simulink library "phaseddetectlib"  (R2015a)
settings: Solver=ode45  StartTime=0.0  StopTime=10.0  RelTol=1e-3
values from neighbouring files (symbols this model uses):
  D = Nsig    [espritdoa.m]    (also in radarvcd.m = sqrt((1 + (2 * zeta ./ sqrt(zeta.^2 + 3)))/3); rootmusicdoa.m = D + conv(noise_eigenvects(:,i),conj(flipud(noise_eigenvects()
undefined symbols (not defined in the file or in its folder): magnitude, physconst
libraries: dspmtrx3 x1, dspsigattribs x1
settings Model: CovSFcnEnable=off  Creator=The MathWorks Inc.  LastModifiedBy=The MathWorks Inc.
settings DebuggingCC: UnderspecifiedInitializationDetection=Classic  MergeDetectMultiDrivingBlocksExec=none  SolverPrmCheckMsg=warning

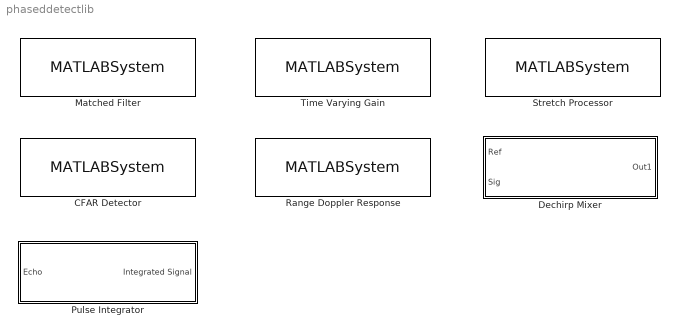
== system phaseddetectlib ==
  CFAR Detector : MATLABSystem  System=phased.CFARDetector  Method=CA  Rank=1  NumGuardCells=2  NumTrainingCells=2  ThresholdFactor=Auto  ProbabilityFalseAlarm=0.1  CustomThresholdFactor=1  ThresholdOutputPort=off  SimulateUsing=Interpreted execution
      mask Type: phased.CFARDetector
      mask Display:
      | disp('CA CFAR');
      | port_label('input',1,'X');
      | port_label('input',2,'Idx');
      | port_label('output',1,'Y');
  Dechirp Mixer : Subsystem  mask(Dechirp){}
      mask help: Mix the input signal with the reference signal. The input signal can be a matrix where each column is a independent channel. The reference signal is a vector. The reference signal is conjugated and then multiplied with each column to compute the output.
      mask Display:
      | port_label('input',1,'RefX');
      | port_label('input',2,'X');
      | port_label('output',1,' ');
      | fprintf('Dechirp')
  Matched Filter : MATLABSystem  System=phased.MatchedFilter  CoefficientsSource=Property  Coefficients=[ 1; 1 ]  SpectrumWindow=None  CustomSpectrumWindow=@hamming  SpectrumRange=[ 0, 1e5 ]  SidelobeAttenuation=30  Beta=0.5  Nbar=4  GainOutputPort=off  SimulateUsing=Interpreted execution
      mask Type: phased.MatchedFilter
      mask Display:
      | disp(['Matched' char(10) 'Filter']);
      | port_label('input',1,'X');
      | port_label('output',1,'Y');
  Pulse Integrator : Subsystem  TreatAsAtomicUnit=on  mask(Pulse Integrator){CoherentFlag=Coherent, N=10, V=0}
      mask prompts: CoherentFlag "Integration method:"; N "Number of pulses to integrate:"; V "Integration overlap (in pulses):"
      mask help: Coherently or noncoherently integrate successive pulses. The input is a column vector representing a pulse. The buffer size, N, specifies how many pulses are integrated. The integration overlap, V, specifies the number of overlapped pulses in successive integrations. V must be less than N.
      mask init:
      | cstr = get_param(gcb,'CoherentFlag');
      | set_param([gcb, '/Integrator'],'OverrideUsingVariant',cstr);
      | validateattributes(N,{'numeric'},{'positive','integer'},'','N');
      | validateattributes(V,{'numeric'},{'integer','>=',0,'<',N},'','K');
      | if strcmp(cstr,'Coherent')
      |     outstr = '\Sigma x';
      | else
      |     outstr = '(\Sigma{|x|^2})^{1/2}';
      | end
      mask TypeOptions CoherentFlag: Coherent | Noncoherent
      mask Display:
      | fprintf('%s\n%d-Pulse\nIntegrator',cstr,N)
      | port_label('input',1,'x');
      | port_label('output',1,outstr,'texmode','on');
  Range Doppler Response : MATLABSystem  System=phased.RangeDopplerResponse  RangeMethod=Matched filter  PropagationSpeed=physconst( 'lightspeed' )  SweepSlope=1e9  DechirpInput=off  RangeFFTLengthSource=Auto  RangeFFTLength=1024  RangeWindow=None  RangeSidelobeAttenuation=30  CustomRangeWindow=@hamming  DopplerFFTLengthSource=Auto  DopplerFFTLength=1024  DopplerWindow=None  DopplerSidelobeAttenuation=30  CustomDopplerWindow=@hamming  DopplerOutput=Frequency  OperatingFrequency=3e8  SimulateUsing=Interpreted execution
      mask Type: phased.RangeDopplerResponse
      mask Display:
      | disp(['Range-Doppler' char(10) 'Response']);
      | port_label('input',1,'X');
      | port_label('input',2,'Coeff');
      | port_label('output',1,'Resp');
      | port_label('output',2,'Range');
      | port_label('output',3,'Dop');
  Stretch Processor : MATLABSystem  System=phased.StretchProcessor  PulseWidth=50e-6  PRF=1e4  SweepSlope=2e9  SweepInterval=Positive  PropagationSpeed=physconst( 'LightSpeed' )  ReferenceRange=5000  RangeSpan=500  SimulateUsing=Interpreted execution
      mask Type: phased.StretchProcessor
      mask Display: disp(['Stretch' char(10) 'Processor']);
  Time Varying Gain : MATLABSystem  System=phased.TimeVaryingGain  RangeLoss=0  ReferenceLoss=0  SimulateUsing=Interpreted execution
      mask Type: phased.TimeVaryingGain
      mask Display: disp('TVG');

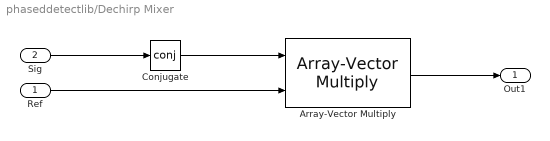
== system phaseddetectlib/Dechirp Mixer ==
  Ref : Inport
  Sig : Inport  Port=2
  Array-Vector Multiply : dspmtrx3/Array-Vector Multiply  mode=Mute  saveAsFlag=0  Dimension=1  V_Source=Input port  V_VectFromMask=[0.5 0.25]  firstCoeffSignedness=Auto  firstCoeffDataTypeStr=Inherit: Same word length as input  firstCoeffLastDataTypeStr=Inherit: Same word length as input  firstCoeffMin=[]  firstCoeffMax=[]  outputSignedness=Auto  outputDataTypeStr=Inherit: Same as product output  outputLastDataTypeStr=Inherit: Same as product output  outputMin=[]  outputMax=[]  accumSignedness=Auto  prodOutputSignedness=Auto  roundingMode=Floor  overflowMode=off
  Conjugate : Math  Operator=conj  SaturateOnIntegerOverflow=on
  Out1 : Outport
  wires:
  Array-Vector Multiply/1 -> Out1/1
  Conjugate/1 -> Array-Vector Multiply/1
  Sig/1 -> Conjugate/1
  Ref/1 -> Array-Vector Multiply/2

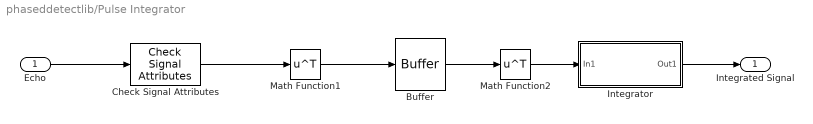
== system phaseddetectlib/Pulse Integrator ==
  Echo : Inport
  Buffer : Buffer  N=N  V=V  TreatMby1Signals=One channel
  Check Signal Attributes : dspsigattribs/Check Signal Attributes  SigAttribCheckMethod=Does not match attributes exactly  Complexity=Ignore  Frame=Ignore  DimsCheckMethod=Is...  Dimensions=Column vector (2-D) or scalar  DatatypeCheckMethod=Ignore  DatatypeGeneral=Boolean  DtypeFloatSpecific=Any floating-point  DtypeFixedSpecific=Any fixed-point  DtypeIntSpecific=Any integer  SampleMode=Ignore
  Integrator : Subsystem  Variant=on  OverrideUsingVariant=Coherent
  Math Function1 : Math  Operator=transpose  OutputSignalType=complex  SaturateOnIntegerOverflow=on
  Math Function2 : Math  Operator=transpose  OutputSignalType=complex  SaturateOnIntegerOverflow=on
  Integrated Signal : Outport
  wires:
  Buffer/1 -> Math Function2/1
  Echo/1 -> Check Signal Attributes/1
  Math Function1/1 -> Buffer/1
  Math Function2/1 -> Integrator/1(In1)
  Integrator/1(Out1) -> Integrated Signal/1
  Check Signal Attributes/1 -> Math Function1/1

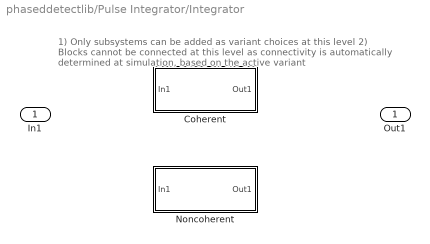
== system phaseddetectlib/Pulse Integrator/Integrator ==
  note: 1) Only subsystems can be added as variant choices at this level
      | 2) Blocks cannot be connected at this level as connectivity is
      | automatically determined at simulation, based on the active variant
  In1 : Inport
  Coherent : Subsystem  VariantControl=Coherent
  Noncoherent : Subsystem  VariantControl=Noncoherent
  Out1 : Outport

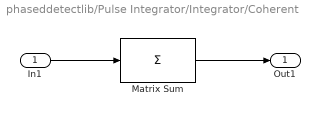
== system phaseddetectlib/Pulse Integrator/Integrator/Coherent ==
  In1 : Inport
  Matrix Sum : Sum  Inputs=+  CollapseMode=Specified dimension  CollapseDim=2
  Out1 : Outport
  wires:
  Matrix Sum/1 -> Out1/1
  In1/1 -> Matrix Sum/1

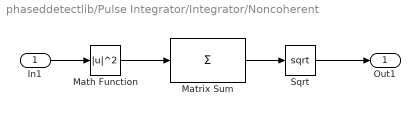
== system phaseddetectlib/Pulse Integrator/Integrator/Noncoherent ==
  In1 : Inport
  Math Function : Math  Operator=magnitude^2  OutputSignalType=real  SaturateOnIntegerOverflow=on
  Matrix Sum : Sum  Inputs=+  CollapseMode=Specified dimension  CollapseDim=2
  Sqrt : Sqrt  OutputSignalType=real  SaturateOnIntegerOverflow=on
  Out1 : Outport
  wires:
  Math Function/1 -> Matrix Sum/1
  In1/1 -> Math Function/1
  Matrix Sum/1 -> Sqrt/1
  Sqrt/1 -> Out1/1
